simulink model "test"  (R2024a)
settings: Solver=VariableStepAuto  StartTime=0.0  StopTime=inf  RelTol=1e-3
undefined symbols (not defined in the file or in its folder): angular, linear
libraries: ros2lib x6
settings Model: Creator=eswarm  LastModifiedBy=eswarm

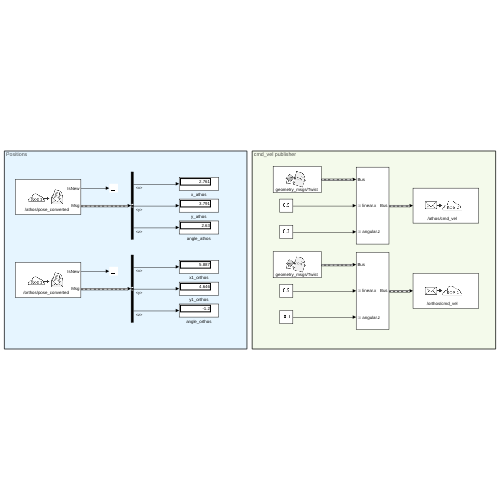
[thumbnail: Simulink's stored preview of the top-level diagram]
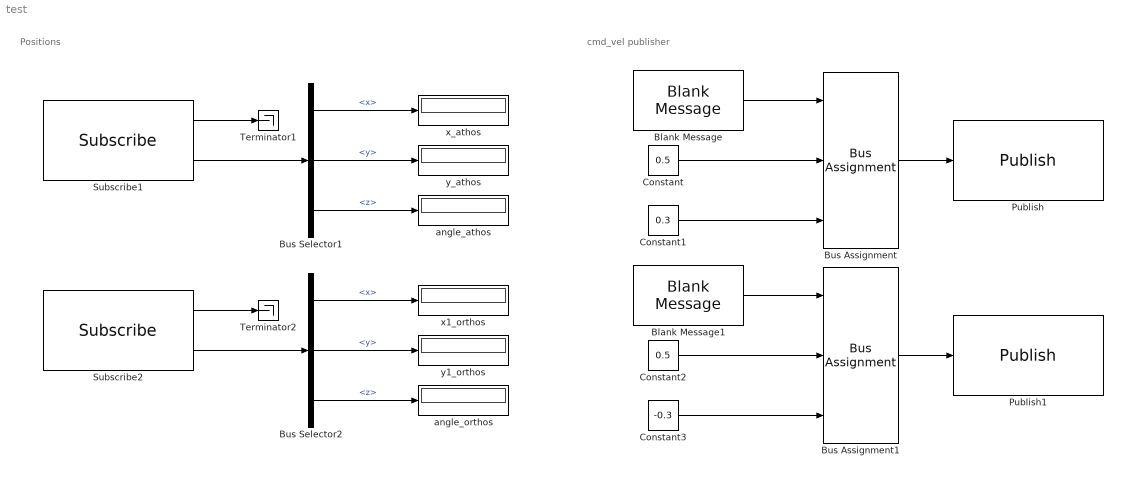
== system test ==
  note: Positions
  note: cmd_vel publisher
  Blank Message : ros2lib/Blank Message  messageClass=Message  entityType=geometry_msgs/Twist  messageType=geometry_msgs/Twist  SampleTime=0.1
  Blank Message1 : ros2lib/Blank Message  messageClass=Message  entityType=geometry_msgs/Twist  messageType=geometry_msgs/Twist  SampleTime=0.1
  Bus Assignment : BusAssignment  AssignedSignals=linear.x,angular.z
  Bus Assignment1 : BusAssignment  AssignedSignals=linear.x,angular.z
  Bus Selector1 : BusSelector  OutputSignals=position.x,position.y,orientation.z
  Bus Selector2 : BusSelector  OutputSignals=position.x,position.y,orientation.z
  Constant : Constant  Value=0.5
  Constant1 : Constant  Value=0.3
  Constant2 : Constant  Value=0.5
  Constant3 : Constant  Value=-0.3
  Publish : ros2lib/Publish  topicSource=Select from ROS network  topic=/athos/cmd_vel  messageType=geometry_msgs/Twist  QOSHistory=Keep last  QOSDepth=1  QOSReliability=Reliable  QOSDurability=Volatile  QOSDeadline=Inf  QOSLifespan=Inf  QOSLiveliness=Automatic  QOSLeaseDuration=Inf  QOSAvoidROSNamespaceConventions=off
  Publish1 : ros2lib/Publish  topicSource=Select from ROS network  topic=/orthos/cmd_vel  messageType=geometry_msgs/Twist  QOSHistory=Keep last  QOSDepth=1  QOSReliability=Reliable  QOSDurability=Volatile  QOSDeadline=Inf  QOSLifespan=Inf  QOSLiveliness=Automatic  QOSLeaseDuration=Inf  QOSAvoidROSNamespaceConventions=off
  Subscribe1 : ros2lib/Subscribe  topicSource=Select from ROS network  topic=/athos/pose_converted  messageType=geometry_msgs/Pose  sampleTime=0.1  QOSHistory=Keep last  QOSDepth=1  QOSReliability=Reliable  QOSDurability=Volatile  QOSDeadline=Inf  QOSLifespan=Inf  QOSLiveliness=Automatic  QOSLeaseDuration=Inf  QOSAvoidROSNamespaceConventions=off
  Subscribe2 : ros2lib/Subscribe  topicSource=Select from ROS network  topic=/orthos/pose_converted  messageType=geometry_msgs/Pose  sampleTime=0.1  QOSHistory=Keep last  QOSDepth=1  QOSReliability=Reliable  QOSDurability=Volatile  QOSDeadline=Inf  QOSLifespan=Inf  QOSLiveliness=Automatic  QOSLeaseDuration=Inf  QOSAvoidROSNamespaceConventions=off
  Terminator1 : Terminator
  Terminator2 : Terminator
  angle_athos : Display
  angle_orthos : Display
  x1_orthos : Display
  x_athos : Display
  y1_orthos : Display
  y_athos : Display
  wires:
  Subscribe1/2 -> Bus Selector1/1
  Subscribe1/1 -> Terminator1/1
  Bus Selector1/1 -> x_athos/1  "<x>"
  Bus Selector1/2 -> y_athos/1  "<y>"
  Bus Selector1/3 -> angle_athos/1  "<z>"
  Bus Selector2/1 -> x1_orthos/1  "<x>"
  Subscribe2/2 -> Bus Selector2/1
  Bus Selector2/3 -> angle_orthos/1  "<z>"
  Subscribe2/1 -> Terminator2/1
  Bus Selector2/2 -> y1_orthos/1  "<y>"
  Bus Assignment/1 -> Publish/1
  Blank Message/1 -> Bus Assignment/1
  Constant/1 -> Bus Assignment/2
  Constant1/1 -> Bus Assignment/3
  Bus Assignment1/1 -> Publish1/1
  Blank Message1/1 -> Bus Assignment1/1
  Constant3/1 -> Bus Assignment1/3
  Constant2/1 -> Bus Assignment1/2
